simulink model "pocket_correlator"  (R2012b)
settings: Solver=ode45  StartTime=0.0  StopTime=10.0  RelTol=1e-3
libraries: xbsIndex_r4 x12697, casper_library_misc x57, simulink x17, casper_library_delays x14, dspsigops x12, xbsReplacements_r4 x10, xps_library x1
(part 4 of 125)

== system pocket_correlator/requant0 ==
  sync : Inport
  gain : Inport  Port=2
  in_even : Inport  Port=3
  in_odd : Inport  Port=4
  Constant{,1..3} (4 alike) : xbsIndex_r4/Constant  const=-1+1/(2^3)  gui_display_data_type=Fixed-point  arith_type=Signed (2's comp)  n_bits=4  bin_pt=3  preci_type=Single  exp_width=8  frac_width=24  explicit_period=on  period=1  equ=P=C  opselect=C  inp2=PCIN>>17  opr=+  inp1=P  carry=CIN  dbl_ovrd=off  block_type=constant
  Delay : xbsIndex_r4/Delay  rst=off  infoeditControl=Selection of Reset will increase slice count due to use of real FFs and instead of SRLs  en=off  latency=2  dbl_ovrd=off  reg_retiming=off  block_type=delay
  Delay1 : xbsIndex_r4/Delay  rst=off  infoeditControl=Selection of Reset will increase slice count due to use of real FFs and instead of SRLs  en=off  latency=3  dbl_ovrd=off  reg_retiming=off  block_type=delay
  Mult{,1..3} (4 alike) : xbsIndex_r4/Mult  precision=Full  arith_type="Signed  (2's comp)"  n_bits=16  bin_pt=14  quantization=Truncate  overflow=Wrap  en=off  latency=3  dbl_ovrd=off  use_behavioral_HDL=off  opt=Speed  use_embedded=on  optimum_pipeline=off  pipeline=on  use_rpm=on  placement_style=Triangular  block_type=mult
  Mux{,1..3} (4 alike) : xbsIndex_r4/Mux  inputs=2  en=off  latency=0  precision=Full  arith_type=Unsigned  n_bits=16  bin_pt=14  quantization=Truncate  overflow=Wrap  dbl_ovrd=off  block_type=mux
  Relational{,1..3} (4 alike) : xbsIndex_r4/Relational  mode=a<b  en=off  latency=2  dbl_ovrd=off  block_type=relational
  c_to_ri : casper_library_misc/c_to_ri  n_bits=18  bin_pt=17
  c_to_ri1 : casper_library_misc/c_to_ri  n_bits=18  bin_pt=17
  convert_of : Subsystem  AncestorBlock=casper_library_misc/convert_of  mask(convert_of){bit_width_i=34, binary_point_i=19, bit_width_o=4, binary_point_o=3, latency=2, overflow=Saturate, quantization=Round  (unbiased: even values)}
      mask prompts: bit_width_i "Bit Width In"; binary_point_i "Binary Point In"; bit_width_o "Bit Width Out"; binary_point_o "Binary Point Out"; overflow "Overflow Behaviour"; quantization "Quantization Behaviour"
      mask help:
      | Converts from one 2's complement bit-width
      | and/or binary point position to another.
      | Includes underflow/overflow indicator.
      mask init:
      | convert_of_init(gcb, ...
      |     'bit_width_i', bit_width_i, ...
      |     'binary_point_i', binary_point_i, ...
      |     'bit_width_o', bit_width_o, ...
      |     'binary_point_o', binary_point_o, ...
      |     'latency', latency, ...
      |     'overflow', overflow, ...
      |     'quantization', quantization);
      settings: AttributesFormatString=[34,19]->[4,3]
      mask TypeOptions overflow: Wrap | Saturate | Error
      mask TypeOptions quantization: Truncate | Round  (unbiased: +/- Inf) | Round  (unbiased: even values)
  convert_of1 : Subsystem  AncestorBlock=casper_library_misc/convert_of  mask(convert_of){bit_width_i=34, binary_point_i=19, bit_width_o=4, binary_point_o=3, latency=2, overflow=Saturate, quantization=Round  (unbiased: even values)}
      mask prompts: bit_width_i "Bit Width In"; binary_point_i "Binary Point In"; bit_width_o "Bit Width Out"; binary_point_o "Binary Point Out"; overflow "Overflow Behaviour"; quantization "Quantization Behaviour"
      mask help:
      | Converts from one 2's complement bit-width
      | and/or binary point position to another.
      | Includes underflow/overflow indicator.
      mask init: same as pocket_correlator/requant0/convert_of
      settings: AttributesFormatString=[34,19]->[4,3]
      mask TypeOptions overflow: Wrap | Saturate | Error
      mask TypeOptions quantization: Truncate | Round  (unbiased: +/- Inf) | Round  (unbiased: even values)
  convert_of2 : Subsystem  AncestorBlock=casper_library_misc/convert_of  mask(convert_of){bit_width_i=34, binary_point_i=19, bit_width_o=4, binary_point_o=3, latency=2, overflow=Saturate, quantization=Round  (unbiased: even values)}
      mask prompts: bit_width_i "Bit Width In"; binary_point_i "Binary Point In"; bit_width_o "Bit Width Out"; binary_point_o "Binary Point Out"; overflow "Overflow Behaviour"; quantization "Quantization Behaviour"
      mask help:
      | Converts from one 2's complement bit-width
      | and/or binary point position to another.
      | Includes underflow/overflow indicator.
      mask init: same as pocket_correlator/requant0/convert_of
      settings: AttributesFormatString=[34,19]->[4,3]
      mask TypeOptions overflow: Wrap | Saturate | Error
      mask TypeOptions quantization: Truncate | Round  (unbiased: +/- Inf) | Round  (unbiased: even values)
  convert_of3 : Subsystem  AncestorBlock=casper_library_misc/convert_of  mask(convert_of){bit_width_i=34, binary_point_i=19, bit_width_o=4, binary_point_o=3, latency=2, overflow=Saturate, quantization=Round  (unbiased: even values)}
      mask prompts: bit_width_i "Bit Width In"; binary_point_i "Binary Point In"; bit_width_o "Bit Width Out"; binary_point_o "Binary Point Out"; overflow "Overflow Behaviour"; quantization "Quantization Behaviour"
      mask help:
      | Converts from one 2's complement bit-width
      | and/or binary point position to another.
      | Includes underflow/overflow indicator.
      mask init: same as pocket_correlator/requant0/convert_of
      settings: AttributesFormatString=[34,19]->[4,3]
      mask TypeOptions overflow: Wrap | Saturate | Error
      mask TypeOptions quantization: Truncate | Round  (unbiased: +/- Inf) | Round  (unbiased: even values)
  ri_to_c : casper_library_misc/ri_to_c
  ri_to_c1 : casper_library_misc/ri_to_c
  sync_out : Outport
  out_even : Outport  Port=2
  out_odd : Outport  Port=3
  wires:
  sync/1 -> [sync_in], Delay1/1
  in_even/1 -> c_to_ri/1
  Mult/1 -> Relational/1, convert_of/1(din)
  Delay/1 -> sync_out/1
  Constant/1 -> Mux/3, Relational/2
  convert_of/1(dout) -> Mux/2
  Mult1/1 -> Relational1/1, convert_of1/1(din)
  Constant1/1 -> Relational1/2, Mux1/3
  convert_of1/1(dout) -> Mux1/2
  Mux/1 -> ri_to_c/1
  Mux1/1 -> ri_to_c/2
  ri_to_c/1 -> out_even/1
  in_odd/1 -> c_to_ri1/1
  Mult2/1 -> convert_of2/1(din), Relational2/1
  Constant2/1 -> Relational2/2, Mux2/3
  convert_of2/1(dout) -> Mux2/2
  Mult3/1 -> Relational3/1, convert_of3/1(din)
  Constant3/1 -> Mux3/3, Relational3/2
  convert_of3/1(dout) -> Mux3/2
  Mux2/1 -> ri_to_c1/1
  Mux3/1 -> ri_to_c1/2
  ri_to_c1/1 -> out_odd/1
  c_to_ri/1 -> Mult/2
  c_to_ri/2 -> Mult1/2
  gain/1 -> Mult2/1, Mult3/1, Mult1/1, Mult/1
  c_to_ri1/1 -> Mult2/2
  c_to_ri1/2 -> Mult3/2
  Delay1/1 -> Delay/1
  convert_of/2(of) -> [of0]
  convert_of1/2(of) -> [of1]
  convert_of2/2(of) -> [of2]
  convert_of3/2(of) -> [of3]
  Relational/1 -> Mux/1
  Relational1/1 -> Mux1/1
  Relational2/1 -> Mux2/1
  Relational3/1 -> Mux3/1

== system pocket_correlator/requant1 ==
  sync : Inport
  gain : Inport  Port=2
  in_even : Inport  Port=3
  in_odd : Inport  Port=4
  Constant{,1..3} (4 alike) : xbsIndex_r4/Constant  const=-1+1/(2^3)  gui_display_data_type=Fixed-point  arith_type=Signed (2's comp)  n_bits=4  bin_pt=3  preci_type=Single  exp_width=8  frac_width=24  explicit_period=on  period=1  equ=P=C  opselect=C  inp2=PCIN>>17  opr=+  inp1=P  carry=CIN  dbl_ovrd=off  block_type=constant
  Delay : xbsIndex_r4/Delay  rst=off  infoeditControl=Selection of Reset will increase slice count due to use of real FFs and instead of SRLs  en=off  latency=2  dbl_ovrd=off  reg_retiming=off  block_type=delay
  Delay1 : xbsIndex_r4/Delay  rst=off  infoeditControl=Selection of Reset will increase slice count due to use of real FFs and instead of SRLs  en=off  latency=3  dbl_ovrd=off  reg_retiming=off  block_type=delay
  Mult{,1..3} (4 alike) : xbsIndex_r4/Mult  precision=Full  arith_type="Signed  (2's comp)"  n_bits=16  bin_pt=14  quantization=Truncate  overflow=Wrap  en=off  latency=3  dbl_ovrd=off  use_behavioral_HDL=off  opt=Speed  use_embedded=on  optimum_pipeline=off  pipeline=on  use_rpm=on  placement_style=Triangular  block_type=mult
  Mux{,1..3} (4 alike) : xbsIndex_r4/Mux  inputs=2  en=off  latency=0  precision=Full  arith_type=Unsigned  n_bits=16  bin_pt=14  quantization=Truncate  overflow=Wrap  dbl_ovrd=off  block_type=mux
  Relational{,1..3} (4 alike) : xbsIndex_r4/Relational  mode=a<b  en=off  latency=2  dbl_ovrd=off  block_type=relational
  c_to_ri : casper_library_misc/c_to_ri  n_bits=18  bin_pt=17
  c_to_ri1 : casper_library_misc/c_to_ri  n_bits=18  bin_pt=17
  convert_of : Subsystem  AncestorBlock=casper_library_misc/convert_of  mask(convert_of){bit_width_i=34, binary_point_i=19, bit_width_o=4, binary_point_o=3, latency=2, overflow=Saturate, quantization=Round  (unbiased: even values)}
      mask prompts: bit_width_i "Bit Width In"; binary_point_i "Binary Point In"; bit_width_o "Bit Width Out"; binary_point_o "Binary Point Out"; overflow "Overflow Behaviour"; quantization "Quantization Behaviour"
      mask help:
      | Converts from one 2's complement bit-width
      | and/or binary point position to another.
      | Includes underflow/overflow indicator.
      mask init: same as pocket_correlator/requant0/convert_of
      settings: AttributesFormatString=[34,19]->[4,3]
      mask TypeOptions overflow: Wrap | Saturate | Error
      mask TypeOptions quantization: Truncate | Round  (unbiased: +/- Inf) | Round  (unbiased: even values)
  convert_of1 : Subsystem  AncestorBlock=casper_library_misc/convert_of  mask(convert_of){bit_width_i=34, binary_point_i=19, bit_width_o=4, binary_point_o=3, latency=2, overflow=Saturate, quantization=Round  (unbiased: even values)}
      mask prompts: bit_width_i "Bit Width In"; binary_point_i "Binary Point In"; bit_width_o "Bit Width Out"; binary_point_o "Binary Point Out"; overflow "Overflow Behaviour"; quantization "Quantization Behaviour"
      mask help:
      | Converts from one 2's complement bit-width
      | and/or binary point position to another.
      | Includes underflow/overflow indicator.
      mask init: same as pocket_correlator/requant0/convert_of
      settings: AttributesFormatString=[34,19]->[4,3]
      mask TypeOptions overflow: Wrap | Saturate | Error
      mask TypeOptions quantization: Truncate | Round  (unbiased: +/- Inf) | Round  (unbiased: even values)
  convert_of2 : Subsystem  AncestorBlock=casper_library_misc/convert_of  mask(convert_of){bit_width_i=34, binary_point_i=19, bit_width_o=4, binary_point_o=3, latency=2, overflow=Saturate, quantization=Round  (unbiased: even values)}
      mask prompts: bit_width_i "Bit Width In"; binary_point_i "Binary Point In"; bit_width_o "Bit Width Out"; binary_point_o "Binary Point Out"; overflow "Overflow Behaviour"; quantization "Quantization Behaviour"
      mask help:
      | Converts from one 2's complement bit-width
      | and/or binary point position to another.
      | Includes underflow/overflow indicator.
      mask init: same as pocket_correlator/requant0/convert_of
      settings: AttributesFormatString=[34,19]->[4,3]
      mask TypeOptions overflow: Wrap | Saturate | Error
      mask TypeOptions quantization: Truncate | Round  (unbiased: +/- Inf) | Round  (unbiased: even values)
  convert_of3 : Subsystem  AncestorBlock=casper_library_misc/convert_of  mask(convert_of){bit_width_i=34, binary_point_i=19, bit_width_o=4, binary_point_o=3, latency=2, overflow=Saturate, quantization=Round  (unbiased: even values)}
      mask prompts: bit_width_i "Bit Width In"; binary_point_i "Binary Point In"; bit_width_o "Bit Width Out"; binary_point_o "Binary Point Out"; overflow "Overflow Behaviour"; quantization "Quantization Behaviour"
      mask help:
      | Converts from one 2's complement bit-width
      | and/or binary point position to another.
      | Includes underflow/overflow indicator.
      mask init: same as pocket_correlator/requant0/convert_of
      settings: AttributesFormatString=[34,19]->[4,3]
      mask TypeOptions overflow: Wrap | Saturate | Error
      mask TypeOptions quantization: Truncate | Round  (unbiased: +/- Inf) | Round  (unbiased: even values)
  ri_to_c : casper_library_misc/ri_to_c
  ri_to_c1 : casper_library_misc/ri_to_c
  sync_out : Outport
  out_even : Outport  Port=2
  out_odd : Outport  Port=3
  wires:
  Relational3/1 -> Mux3/1
  Relational2/1 -> Mux2/1
  Relational1/1 -> Mux1/1
  Relational/1 -> Mux/1
  convert_of3/2(of) -> [of3]
  convert_of2/2(of) -> [of2]
  convert_of1/2(of) -> [of1]
  convert_of/2(of) -> [of0]
  Delay1/1 -> Delay/1
  c_to_ri1/2 -> Mult3/2
  c_to_ri1/1 -> Mult2/2
  gain/1 -> Mult/1, Mult1/1, Mult3/1, Mult2/1
  c_to_ri/2 -> Mult1/2
  c_to_ri/1 -> Mult/2
  ri_to_c1/1 -> out_odd/1
  Mux3/1 -> ri_to_c1/2
  Mux2/1 -> ri_to_c1/1
  convert_of3/1(dout) -> Mux3/2
  Constant3/1 -> Relational3/2, Mux3/3
  Mult3/1 -> convert_of3/1(din), Relational3/1
  convert_of2/1(dout) -> Mux2/2
  Constant2/1 -> Mux2/3, Relational2/2
  Mult2/1 -> Relational2/1, convert_of2/1(din)
  in_odd/1 -> c_to_ri1/1
  ri_to_c/1 -> out_even/1
  Mux1/1 -> ri_to_c/2
  Mux/1 -> ri_to_c/1
  convert_of1/1(dout) -> Mux1/2
  Constant1/1 -> Mux1/3, Relational1/2
  Mult1/1 -> convert_of1/1(din), Relational1/1
  convert_of/1(dout) -> Mux/2
  Constant/1 -> Relational/2, Mux/3
  Delay/1 -> sync_out/1
  Mult/1 -> convert_of/1(din), Relational/1
  in_even/1 -> c_to_ri/1
  sync/1 -> Delay1/1, [sync_in]

== system pocket_correlator/sync_ctrl ==
  sim_1 : Inport
  sim_2 : Inport  Port=2
  sim_3 : Inport  Port=3
  convert1_1 : DataTypeConversion  OutDataTypeStr=fixdt('ufix1_En0')  LockScale=on
  convert1_2 : DataTypeConversion  OutDataTypeStr=fixdt('ufix1_En0')  LockScale=on
  convert1_3 : DataTypeConversion  OutDataTypeStr=fixdt('ufix1_En0')  LockScale=on
  convert2_1 : DataTypeConversion  OutDataTypeStr=fixdt('ufix1_En0')  ConvertRealWorld=Stored Integer (SI)  LockScale=on
  convert2_2 : DataTypeConversion  OutDataTypeStr=fixdt('ufix1_En0')  ConvertRealWorld=Stored Integer (SI)  LockScale=on
  convert2_3 : DataTypeConversion  OutDataTypeStr=fixdt('ufix1_En0')  ConvertRealWorld=Stored Integer (SI)  LockScale=on
  gain_1 : Gain  Gain=4
  gain_2 : Gain  Gain=2
  gain_3 : Gain
  io_delay : xbsIndex_r4/Delay  rst=off  infoeditControl=Selection of Reset will increase slice count due to use of real FFs and instead of SRLs  en=off  latency=0  dbl_ovrd=off  reg_retiming=on  block_type=delay
  pocket_correlator_sync_ctrl_user_data_out : xbsIndex_r4/Gateway In  gui_display_data_type=Fixed-point  arith_type=Unsigned  n_bits=32  bin_pt=0  preci_type=Single  exp_width=8  frac_width=24  quantization="Round  (unbiased: +/- Inf)"  overflow=Saturate  period=1  dbl_ovrd=off  timing_constraint=None  locs_specified=off  LOCs={}  UseAsADC=off  ADCChannel='1'  inherit_from_input=off  hdl_port=on  block_type=gatewayin
  sim_add : Sum  Inputs=+++  OutDataTypeStr=uint32
  slice_enable_sync : xbsIndex_r4/Slice  nbits=1  boolean_output=on  mode=Lower Bit Location + Width  bit1=0  base1=MSB of Input  bit0=2  base0=LSB of Input  dbl_ovrd=off  block_type=slice
  slice_master_reset : xbsIndex_r4/Slice  nbits=1  boolean_output=on  mode=Lower Bit Location + Width  bit1=0  base1=MSB of Input  bit0=0  base0=LSB of Input  dbl_ovrd=off  block_type=slice
  slice_use_self_pps : xbsIndex_r4/Slice  nbits=1  boolean_output=on  mode=Lower Bit Location + Width  bit1=0  base1=MSB of Input  bit0=1  base0=LSB of Input  dbl_ovrd=off  block_type=slice
  in_enable_sync : Outport
  in_use_self_pps : Outport  Port=2
  in_master_reset : Outport  Port=3
  wires:
  pocket_correlator_sync_ctrl_user_data_out/1 -> io_delay/1
  sim_add/1 -> pocket_correlator_sync_ctrl_user_data_out/1
  sim_1/1 -> convert1_1/1
  convert1_1/1 -> convert2_1/1
  convert2_1/1 -> gain_1/1
  gain_1/1 -> sim_add/1
  io_delay/1 -> slice_enable_sync/1, slice_use_self_pps/1, slice_master_reset/1
  slice_enable_sync/1 -> in_enable_sync/1
  sim_2/1 -> convert1_2/1
  convert1_2/1 -> convert2_2/1
  convert2_2/1 -> gain_2/1
  gain_2/1 -> sim_add/2
  slice_use_self_pps/1 -> in_use_self_pps/1
  sim_3/1 -> convert1_3/1
  convert1_3/1 -> convert2_3/1
  convert2_3/1 -> gain_3/1
  gain_3/1 -> sim_add/3
  slice_master_reset/1 -> in_master_reset/1

== system pocket_correlator/acc_ctrl/edge_detect ==
  in : Inport
  Delay : xbsIndex_r4/Delay  rst=off  infoeditControl=Selection of Reset will increase slice count due to use of real FFs and instead of SRLs  en=off  latency=1  dbl_ovrd=off  reg_retiming=off  block_type=delay
      settings: xl_area=[0, 0, 0, 0, 0, 0, 0]
  Inverter : xbsIndex_r4/Inverter  en=off  latency=0  dbl_ovrd=off  block_type=inv
      settings: xl_area=[0, 0, 0, 0, 0, 0, 0]
  edge_op : xbsIndex_r4/Logical  logical_function=NOR  inputs=2  en=off  latency=0  precision=Full  arith_type=Unsigned  n_bits=8  bin_pt=2  align_bp=on  dbl_ovrd=off  block_type=logical
      settings: xl_area=[0, 0, 0, 0, 0, 0, 0]
  out : Outport
  wires:
  Inverter/1 -> edge_op/1
  edge_op/1 -> out/1
  in/1 -> Inverter/1, Delay/1
  Delay/1 -> edge_op/2

== system pocket_correlator/acc_ctrl/edge_detect1 ==
  in : Inport
  Delay : xbsIndex_r4/Delay  rst=off  infoeditControl=Selection of Reset will increase slice count due to use of real FFs and instead of SRLs  en=off  latency=1  dbl_ovrd=off  reg_retiming=off  block_type=delay
      settings: xl_area=[0, 0, 0, 0, 0, 0, 0]
  Inverter : xbsIndex_r4/Inverter  en=off  latency=0  dbl_ovrd=off  block_type=inv
      settings: xl_area=[0, 0, 0, 0, 0, 0, 0]
  edge_op : xbsIndex_r4/Logical  logical_function=NOR  inputs=2  en=off  latency=0  precision=Full  arith_type=Unsigned  n_bits=8  bin_pt=2  align_bp=on  dbl_ovrd=off  block_type=logical
      settings: xl_area=[0, 0, 0, 0, 0, 0, 0]
  out : Outport
  wires:
  Inverter/1 -> edge_op/1
  edge_op/1 -> out/1
  in/1 -> Inverter/1, Delay/1
  Delay/1 -> edge_op/2

== system pocket_correlator/acc_ctrl/edge_detect2 ==
  in : Inport
  Delay : xbsIndex_r4/Delay  rst=off  infoeditControl=Selection of Reset will increase slice count due to use of real FFs and instead of SRLs  en=off  latency=1  dbl_ovrd=off  reg_retiming=off  block_type=delay
      settings: xl_area=[0, 0, 0, 0, 0, 0, 0]
  Inverter : xbsIndex_r4/Inverter  en=off  latency=0  dbl_ovrd=off  block_type=inv
      settings: xl_area=[0, 0, 0, 0, 0, 0, 0]
  edge_op : xbsIndex_r4/Logical  logical_function=NOR  inputs=2  en=off  latency=0  precision=Full  arith_type=Unsigned  n_bits=8  bin_pt=2  align_bp=on  dbl_ovrd=off  block_type=logical
      settings: xl_area=[0, 0, 0, 0, 0, 0, 0]
  out : Outport
  wires:
  Inverter/1 -> edge_op/1
  edge_op/1 -> out/1
  in/1 -> Inverter/1, Delay/1
  Delay/1 -> edge_op/2

== system pocket_correlator/calc_adc_sum_sq/edge_detect2 ==
  in : Inport
  Delay : xbsIndex_r4/Delay  rst=off  infoeditControl=Selection of Reset will increase slice count due to use of real FFs and instead of SRLs  en=off  latency=1  dbl_ovrd=off  reg_retiming=off  block_type=delay
      settings: xl_area=[0, 0, 0, 0, 0, 0, 0]
  Inverter : xbsIndex_r4/Inverter  en=off  latency=0  dbl_ovrd=off  block_type=inv
      settings: xl_area=[0, 0, 0, 0, 0, 0, 0]
  edge_op : xbsIndex_r4/Logical  logical_function=AND  inputs=2  en=off  latency=0  precision=Full  arith_type=Unsigned  n_bits=8  bin_pt=2  align_bp=on  dbl_ovrd=off  block_type=logical
      settings: xl_area=[0, 0, 0, 0, 0, 0, 0]
  out : Outport
  wires:
  Inverter/1 -> edge_op/1
  edge_op/1 -> out/1
  in/1 -> Inverter/1, Delay/1
  Delay/1 -> edge_op/2

== system pocket_correlator/calc_adc_sum_sq4/edge_detect2 ==
  in : Inport
  Delay : xbsIndex_r4/Delay  rst=off  infoeditControl=Selection of Reset will increase slice count due to use of real FFs and instead of SRLs  en=off  latency=1  dbl_ovrd=off  reg_retiming=off  block_type=delay
      settings: xl_area=[0, 0, 0, 0, 0, 0, 0]
  Inverter : xbsIndex_r4/Inverter  en=off  latency=0  dbl_ovrd=off  block_type=inv
      settings: xl_area=[0, 0, 0, 0, 0, 0, 0]
  edge_op : xbsIndex_r4/Logical  logical_function=AND  inputs=2  en=off  latency=0  precision=Full  arith_type=Unsigned  n_bits=8  bin_pt=2  align_bp=on  dbl_ovrd=off  block_type=logical
      settings: xl_area=[0, 0, 0, 0, 0, 0, 0]
  out : Outport
  wires:
  Inverter/1 -> edge_op/1
  edge_op/1 -> out/1
  in/1 -> Inverter/1, Delay/1
  Delay/1 -> edge_op/2

== system pocket_correlator/dir_x0/aa ==
  a+bi : Inport
  c+di : Inport  Port=2
  new_acc : Inport  Port=3
  Counter : xbsIndex_r4/Counter  cnt_type=Free Running  cnt_to=Inf  operation=Up  start_count=0  cnt_by_val=1  arith_type=Unsigned  n_bits=chan_bits  bin_pt=0  load_pin=off  rst=on  en=on  explicit_period=off  period=1  dbl_ovrd=off  use_behavioral_HDL=off  implementation=Fabric  use_rpm=on  block_type=counter
      settings: xl_area=[0, 0, 0, 0, 0, 0, 0]
  Delay3 : xbsIndex_r4/Delay  rst=off  infoeditControl=Selection of Reset will increase slice count due to use of real FFs and instead of SRLs  en=off  latency=4  dbl_ovrd=off  reg_retiming=off  block_type=delay
      settings: xl_area=[0, 0, 0, 0, 0, 0, 0]
  Gateway Out{,1..3} (4 alike) : xbsIndex_r4/Gateway Out  inherit_from_input=off  hdl_port=on  timing_constraint=None  locs_specified=off  LOCs={}  UseAsDAC=off  DACChannel='1'  block_type=gatewayout
      settings: infoedit="Gateway out block.  Converts Xilinx fixed point inputs into ouputs of type Simulink integer, double, or fixed point.<P><P>Hardware notes:  In hardware these blocks become top level output ports or are discarded, depending on how they are configured."  xl_area=[0, 0, 0, 0, 0, 0, 0]  block_version=10.1.3
  Reinterpret : xbsIndex_r4/Reinterpret  force_arith_type=on  arith_type=Unsigned  force_bin_pt=on  bin_pt=0  block_type=reinterpret
      settings: infoedit="Changes signal type without altering the binary representation.   You can changed the signal between signed and unsigned, and relocate the binary point.<P><P>Hardware notes: In hardware this block costs nothing.<P><P>Example:  Suppose the input is 6 bits wide, signed, with 2 fractional bits, and the output is forced to unsigned with 0 fractional bits.  Then an input of -2.0 (1110.00 in binary 2's complement) becomes an output of 56 (111000 in binary)."  block_version=10.1.3
  Scope : Scope  NumInputPorts=4
      settings: YMin=-1~-1~-1~-1  YMax=1~1~1~1
  Terminator : Terminator
  c_to_ri : Subsystem  mask(Complex to Real-Imag){n_bits=4, bin_pt=3}
      mask prompts: n_bits "Bit Width"; bin_pt "Binary Point"
      mask help: Outputs real and imaginary components of a complex input.
      mask init:
      | annotation=sprintf('%d_%d r/i',n_bits,bin_pt);
      | set_param(gcb,'AttributesFormatString',annotation);
      settings: AttributesFormatString=4_3 r/i
      mask Help:
      | <pre>
      | Description::
      | 
      | Outputs real and imaginary components of a complex input.
      | Useful for simplifying interconnects.
      | See also: Real-Imag to Complex (ri_to_c)
      | 
      | Mask Parameters::
      | 
      | Bit Width (n_bits): Specifies the width of the real/imaginary components.
      | Assumed equal for both components.
      | 
      | Binary Point (bin_pt): Specifies the binary point location in the real/imaginary components.
      | Assumed equal for both components.
      | </pre>
  c_to_ri1 : Subsystem  mask(Complex to Real-Imag){n_bits=4, bin_pt=3}
      mask prompts: n_bits "Bit Width"; bin_pt "Binary Point"
      mask help: Outputs real and imaginary components of a complex input.
      mask init:
      | annotation=sprintf('%d_%d r/i',n_bits,bin_pt);
      | set_param(gcb,'AttributesFormatString',annotation);
      settings: AttributesFormatString=4_3 r/i
      mask Help:
      | <pre>
      | Description::
      | 
      | Outputs real and imaginary components of a complex input.
      | Useful for simplifying interconnects.
      | See also: Real-Imag to Complex (ri_to_c)
      | 
      | Mask Parameters::
      | 
      | Bit Width (n_bits): Specifies the width of the real/imaginary components.
      | Assumed equal for both components.
      | 
      | Binary Point (bin_pt): Specifies the binary point location in the real/imaginary components.
      | Assumed equal for both components.
      | </pre>
  cmult_dsp48e : Subsystem  AncestorBlock=casper_library_multipliers/cmult_dsp48e  mask(cmult_dsp48e){n_bits_a=4, bin_pt_a=3, n_bits_b=4, bin_pt_b=3, conjugated=on, full_precision=on, n_bits_c=37, bin_pt_c=34, quantization=Truncate, overflow=Wrap, cast_latency=0}
      mask prompts: n_bits_a "Bit width 'a'"; bin_pt_a "Binary point 'a'"; n_bits_b "Bit width 'b'"; bin_pt_b "Binary point 'b'"; conjugated "Conjugate"; full_precision "Full precision"; n_bits_c "Bit width out"; bin_pt_c "Binary point out"; cast_latency "Cast Latency"
      mask help:
      | Multiplies two complex numbers using 4 DSP48Es.
      | Conjugation is optional.
      |
      | Re{a} and Im{a} can be up to 25 bits.
      | Re{b} and Im{b} can be up to 18 bits.
      mask init:
      | cmult_dsp48e_init(gcb, ...
      |     'n_bits_a', n_bits_a, ...
      |     'bin_pt_a', bin_pt_a, ...
      |     'n_bits_b', n_bits_b, ...
      |     'bin_pt_b', bin_pt_b, ...
      |     'conjugated', conjugated, ...
      |     'full_precision', full_precision, ...
      |     'n_bits_c', n_bits_c, ...
      |     'bin_pt_c', bin_pt_c, ...
      |     'quantization', quantization, ...
      |     'overflow', overflow, ...
      |     'cast_latency', cast_latency);
      settings: AttributesFormatString=|
      | 4_3 * 4_3 ==> 9_6
      | Latency=4
      mask Callback full_precision:
      | full_precision = get_param(gcb, 'full_precision');
      | 
      | if strcmp(full_precision, 'on'),
      |     not_full_precision = 'off';
      | else
      |     not_full_precision = 'on';
      | end
      | 
      | set_param_state(gcb, 'n_bits_c', not_full_precision);
      | set_param_state(gcb, 'bin_pt_c', not_full_precision);
      | set_param_state(gcb, 'quantization', not_full_precision);
      | set_param_state(gcb, 'overflow', not_full_precision);
      | set_param_state(gcb, 'cast_latency', not_full_precision);
      mask TypeOptions quantization: Truncate | Round  (unbiased: +/- Inf) | Round  (unbiased: Even Values)
      mask TypeOptions overflow: Wrap | Saturate | Flag as error
  real : Subsystem  Tag=xps:bram  AncestorBlock=xps_library/Shared BRAM  mask{arith_type=Unsigned, addr_width=max(chan_bits,10), data_width=32, reg_prim_output=off, reg_core_output=off, optimization=Minimum_Area, data_bin_pt=0, init_vals=0, sample_rate=1}
      mask prompts: arith_type "Output Data Type"; addr_width "Address width"; data_width "Data Width"; reg_prim_output "Register Primitive Output"; reg_core_output "Register Core Output"; data_bin_pt "Data Binary Point"; init_vals "Initial values (simulation only)"; sample_rate "Sample rate"
      mask init:
      | shared_bram_mask;
      mask TypeOptions arith_type: Unsigned | Signed  (2's comp)
      mask TypeOptions data_width: 8 | 16 | 32 | 64 | 128
      mask TypeOptions optimization: Minimum_Area | Low_Power
  vacc_32bit : Subsystem  mask{n_chans=n_chans}
      mask prompts: n_chans "Number of channels"
      mask init:
      | chan_bits=ceil(log2(n_chans));
  wires:
  Reinterpret/1 -> real/2(data_in), Gateway Out1/1
  Counter/1 -> real/1(addr), Gateway Out/1
  vacc_32bit/2(valid) -> Counter/2, real/3(we), Gateway Out2/1
  Delay3/1 -> Counter/1, vacc_32bit/2(new_acc), Gateway Out3/1
  c+di/1 -> c_to_ri1/1(c)
  a+bi/1 -> c_to_ri/1(c)
  c_to_ri1/2(im) -> cmult_dsp48e/4(b_im)
  c_to_ri1/1(re) -> cmult_dsp48e/3(b_re)
  c_to_ri/2(im) -> cmult_dsp48e/2(a_im)
  c_to_ri/1(re) -> cmult_dsp48e/1(a_re)
  vacc_32bit/1(dout) -> Reinterpret/1
  new_acc/1 -> Delay3/1
  cmult_dsp48e/1(c_re) -> vacc_32bit/1(din)
  real/1(data_out) -> Terminator/1
  Gateway Out/1 -> Scope/1
  Gateway Out1/1 -> Scope/2
  Gateway Out2/1 -> Scope/3
  Gateway Out3/1 -> Scope/4

== system pocket_correlator/dir_x0/ab ==
  a+bi : Inport
  c+di : Inport  Port=2
  new_acc : Inport  Port=3
  Counter : xbsIndex_r4/Counter  cnt_type=Free Running  cnt_to=Inf  operation=Up  start_count=0  cnt_by_val=1  arith_type=Unsigned  n_bits=11  bin_pt=0  load_pin=off  rst=on  en=on  explicit_period=off  period=1  dbl_ovrd=off  use_behavioral_HDL=off  implementation=Fabric  use_rpm=on  block_type=counter
      settings: xl_area=[0, 0, 0, 0, 0, 0, 0]
  Delay3 : xbsIndex_r4/Delay  rst=off  infoeditControl=Selection of Reset will increase slice count due to use of real FFs and instead of SRLs  en=off  latency=4  dbl_ovrd=off  reg_retiming=off  block_type=delay
      settings: xl_area=[0, 0, 0, 0, 0, 0, 0]
  Reinterpret : xbsIndex_r4/Reinterpret  force_arith_type=on  arith_type=Unsigned  force_bin_pt=on  bin_pt=0  block_type=reinterpret
      settings: infoedit="Changes signal type without altering the binary representation.   You can changed the signal between signed and unsigned, and relocate the binary point.<P><P>Hardware notes: In hardware this block costs nothing.<P><P>Example:  Suppose the input is 6 bits wide, signed, with 2 fractional bits, and the output is forced to unsigned with 0 fractional bits.  Then an input of -2.0 (1110.00 in binary 2's complement) becomes an output of 56 (111000 in binary)."  block_version=10.1.3
  Reinterpret1 : xbsIndex_r4/Reinterpret  force_arith_type=on  arith_type=Unsigned  force_bin_pt=on  bin_pt=0  block_type=reinterpret
      settings: infoedit="Changes signal type without altering the binary representation.   You can changed the signal between signed and unsigned, and relocate the binary point.<P><P>Hardware notes: In hardware this block costs nothing.<P><P>Example:  Suppose the input is 6 bits wide, signed, with 2 fractional bits, and the output is forced to unsigned with 0 fractional bits.  Then an input of -2.0 (1110.00 in binary 2's complement) becomes an output of 56 (111000 in binary)."  block_version=10.1.3
  c_to_ri : Subsystem  mask(Complex to Real-Imag){n_bits=4, bin_pt=3}
      mask prompts: n_bits "Bit Width"; bin_pt "Binary Point"
      mask help: Outputs real and imaginary components of a complex input.
      mask init:
      | annotation=sprintf('%d_%d r/i',n_bits,bin_pt);
      | set_param(gcb,'AttributesFormatString',annotation);
      settings: AttributesFormatString=4_3 r/i
      mask Help:
      | <pre>
      | Description::
      | 
      | Outputs real and imaginary components of a complex input.
      | Useful for simplifying interconnects.
      | See also: Real-Imag to Complex (ri_to_c)
      | 
      | Mask Parameters::
      | 
      | Bit Width (n_bits): Specifies the width of the real/imaginary components.
      | Assumed equal for both components.
      | 
      | Binary Point (bin_pt): Specifies the binary point location in the real/imaginary components.
      | Assumed equal for both components.
      | </pre>
  c_to_ri1 : Subsystem  mask(Complex to Real-Imag){n_bits=4, bin_pt=3}
      mask prompts: n_bits "Bit Width"; bin_pt "Binary Point"
      mask help: Outputs real and imaginary components of a complex input.
      mask init:
      | annotation=sprintf('%d_%d r/i',n_bits,bin_pt);
      | set_param(gcb,'AttributesFormatString',annotation);
      settings: AttributesFormatString=4_3 r/i
      mask Help:
      | <pre>
      | Description::
      | 
      | Outputs real and imaginary components of a complex input.
      | Useful for simplifying interconnects.
      | See also: Real-Imag to Complex (ri_to_c)
      | 
      | Mask Parameters::
      | 
      | Bit Width (n_bits): Specifies the width of the real/imaginary components.
      | Assumed equal for both components.
      | 
      | Binary Point (bin_pt): Specifies the binary point location in the real/imaginary components.
      | Assumed equal for both components.
      | </pre>
  cmult_dsp48e : Subsystem  AncestorBlock=casper_library_multipliers/cmult_dsp48e  mask(cmult_dsp48e){n_bits_a=4, bin_pt_a=3, n_bits_b=4, bin_pt_b=3, conjugated=on, full_precision=on, n_bits_c=37, bin_pt_c=34, quantization=Truncate, overflow=Wrap, cast_latency=0}
      mask prompts: n_bits_a "Bit width 'a'"; bin_pt_a "Binary point 'a'"; n_bits_b "Bit width 'b'"; bin_pt_b "Binary point 'b'"; conjugated "Conjugate"; full_precision "Full precision"; n_bits_c "Bit width out"; bin_pt_c "Binary point out"; cast_latency "Cast Latency"
      mask help:
      | Multiplies two complex numbers using 4 DSP48Es.
      | Conjugation is optional.
      |
      | Re{a} and Im{a} can be up to 25 bits.
      | Re{b} and Im{b} can be up to 18 bits.
      mask init: same as pocket_correlator/dir_x0/aa/cmult_dsp48e
      settings: AttributesFormatString=|
      | 4_3 * 4_3 ==> 9_6
      | Latency=4
      mask Callback full_precision:
      | full_precision = get_param(gcb, 'full_precision');
      | 
      | if strcmp(full_precision, 'on'),
      |     not_full_precision = 'off';
      | else
      |     not_full_precision = 'on';
      | end
      | 
      | set_param_state(gcb, 'n_bits_c', not_full_precision);
      | set_param_state(gcb, 'bin_pt_c', not_full_precision);
      | set_param_state(gcb, 'quantization', not_full_precision);
      | set_param_state(gcb, 'overflow', not_full_precision);
      | set_param_state(gcb, 'cast_latency', not_full_precision);
      mask TypeOptions quantization: Truncate | Round  (unbiased: +/- Inf) | Round  (unbiased: Even Values)
      mask TypeOptions overflow: Wrap | Saturate | Flag as error
  imag : Subsystem  Tag=xps:bram  AncestorBlock=xps_library/Shared BRAM  mask{arith_type=Unsigned, addr_width=max(chan_bits,10), data_width=32, reg_prim_output=off, reg_core_output=off, optimization=Minimum_Area, data_bin_pt=0, init_vals=0, sample_rate=1}
      mask prompts: arith_type "Output Data Type"; addr_width "Address width"; data_width "Data Width"; reg_prim_output "Register Primitive Output"; reg_core_output "Register Core Output"; data_bin_pt "Data Binary Point"; init_vals "Initial values (simulation only)"; sample_rate "Sample rate"
      mask init:
      | shared_bram_mask;
      mask TypeOptions arith_type: Unsigned | Signed  (2's comp)
      mask TypeOptions data_width: 8 | 16 | 32 | 64 | 128
      mask TypeOptions optimization: Minimum_Area | Low_Power
  real : Subsystem  Tag=xps:bram  AncestorBlock=xps_library/Shared BRAM  mask{arith_type=Unsigned, addr_width=max(chan_bits,10), data_width=32, reg_prim_output=off, reg_core_output=off, optimization=Minimum_Area, data_bin_pt=0, init_vals=0, sample_rate=1}
      mask prompts: arith_type "Output Data Type"; addr_width "Address width"; data_width "Data Width"; reg_prim_output "Register Primitive Output"; reg_core_output "Register Core Output"; data_bin_pt "Data Binary Point"; init_vals "Initial values (simulation only)"; sample_rate "Sample rate"
      mask init:
      | shared_bram_mask;
      mask TypeOptions arith_type: Unsigned | Signed  (2's comp)
      mask TypeOptions data_width: 8 | 16 | 32 | 64 | 128
      mask TypeOptions optimization: Minimum_Area | Low_Power
  vacc_0 : Subsystem  mask{n_chans=n_chans}
      mask prompts: n_chans "Number of channels"
      mask init:
      | chan_bits=ceil(log2(n_chans));
  vacc_1 : Subsystem  mask{n_chans=n_chans}
      mask prompts: n_chans "Number of channels"
      mask init:
      | chan_bits=ceil(log2(n_chans));
  wires:
  Counter/1 -> real/1(addr), imag/1(addr)
  vacc_1/1(dout) -> Reinterpret1/1
  Reinterpret1/1 -> imag/2(data_in)
  vacc_1/2(valid) -> imag/3(we)
  Reinterpret/1 -> real/2(data_in)
  vacc_0/2(valid) -> real/3(we), Counter/2
  vacc_0/1(dout) -> Reinterpret/1
  new_acc/1 -> Delay3/1
  Delay3/1 -> vacc_0/2(new_acc), Counter/1, vacc_1/2(new_acc)
  c+di/1 -> c_to_ri1/1(c)
  a+bi/1 -> c_to_ri/1(c)
  c_to_ri1/2(im) -> cmult_dsp48e/4(b_im)
  c_to_ri1/1(re) -> cmult_dsp48e/3(b_re)
  c_to_ri/2(im) -> cmult_dsp48e/2(a_im)
  c_to_ri/1(re) -> cmult_dsp48e/1(a_re)
  cmult_dsp48e/2(c_im) -> vacc_1/1(din)
  cmult_dsp48e/1(c_re) -> vacc_0/1(din)

== system pocket_correlator/dir_x0/bb ==
  a+bi : Inport
  c+di : Inport  Port=2
  new_acc : Inport  Port=3
  Counter : xbsIndex_r4/Counter  cnt_type=Free Running  cnt_to=Inf  operation=Up  start_count=0  cnt_by_val=1  arith_type=Unsigned  n_bits=chan_bits  bin_pt=0  load_pin=off  rst=on  en=on  explicit_period=off  period=1  dbl_ovrd=off  use_behavioral_HDL=off  implementation=Fabric  use_rpm=on  block_type=counter
      settings: xl_area=[0, 0, 0, 0, 0, 0, 0]
  Delay3 : xbsIndex_r4/Delay  rst=off  infoeditControl=Selection of Reset will increase slice count due to use of real FFs and instead of SRLs  en=off  latency=4  dbl_ovrd=off  reg_retiming=off  block_type=delay
      settings: xl_area=[0, 0, 0, 0, 0, 0, 0]
  Gateway Out{,1..3} (4 alike) : xbsIndex_r4/Gateway Out  inherit_from_input=off  hdl_port=on  timing_constraint=None  locs_specified=off  LOCs={}  UseAsDAC=off  DACChannel='1'  block_type=gatewayout
      settings: infoedit="Gateway out block.  Converts Xilinx fixed point inputs into ouputs of type Simulink integer, double, or fixed point.<P><P>Hardware notes:  In hardware these blocks become top level output ports or are discarded, depending on how they are configured."  xl_area=[0, 0, 0, 0, 0, 0, 0]  block_version=10.1.3
  Reinterpret : xbsIndex_r4/Reinterpret  force_arith_type=on  arith_type=Unsigned  force_bin_pt=on  bin_pt=0  block_type=reinterpret
      settings: infoedit="Changes signal type without altering the binary representation.   You can changed the signal between signed and unsigned, and relocate the binary point.<P><P>Hardware notes: In hardware this block costs nothing.<P><P>Example:  Suppose the input is 6 bits wide, signed, with 2 fractional bits, and the output is forced to unsigned with 0 fractional bits.  Then an input of -2.0 (1110.00 in binary 2's complement) becomes an output of 56 (111000 in binary)."  block_version=10.1.3
  Scope : Scope  NumInputPorts=4
      settings: YMin=-1~-1~-1~-1  YMax=1~1~1~1
  Terminator : Terminator
  c_to_ri : Subsystem  mask(Complex to Real-Imag){n_bits=4, bin_pt=3}
      mask prompts: n_bits "Bit Width"; bin_pt "Binary Point"
      mask help: Outputs real and imaginary components of a complex input.
      mask init:
      | annotation=sprintf('%d_%d r/i',n_bits,bin_pt);
      | set_param(gcb,'AttributesFormatString',annotation);
      settings: AttributesFormatString=4_3 r/i
      mask Help:
      | <pre>
      | Description::
      | 
      | Outputs real and imaginary components of a complex input.
      | Useful for simplifying interconnects.
      | See also: Real-Imag to Complex (ri_to_c)
      | 
      | Mask Parameters::
      | 
      | Bit Width (n_bits): Specifies the width of the real/imaginary components.
      | Assumed equal for both components.
      | 
      | Binary Point (bin_pt): Specifies the binary point location in the real/imaginary components.
      | Assumed equal for both components.
      | </pre>
  c_to_ri1 : Subsystem  mask(Complex to Real-Imag){n_bits=4, bin_pt=3}
      mask prompts: n_bits "Bit Width"; bin_pt "Binary Point"
      mask help: Outputs real and imaginary components of a complex input.
      mask init:
      | annotation=sprintf('%d_%d r/i',n_bits,bin_pt);
      | set_param(gcb,'AttributesFormatString',annotation);
      settings: AttributesFormatString=4_3 r/i
      mask Help:
      | <pre>
      | Description::
      | 
      | Outputs real and imaginary components of a complex input.
      | Useful for simplifying interconnects.
      | See also: Real-Imag to Complex (ri_to_c)
      | 
      | Mask Parameters::
      | 
      | Bit Width (n_bits): Specifies the width of the real/imaginary components.
      | Assumed equal for both components.
      | 
      | Binary Point (bin_pt): Specifies the binary point location in the real/imaginary components.
      | Assumed equal for both components.
      | </pre>
  cmult_dsp48e : Subsystem  AncestorBlock=casper_library_multipliers/cmult_dsp48e  mask(cmult_dsp48e){n_bits_a=4, bin_pt_a=3, n_bits_b=4, bin_pt_b=3, conjugated=on, full_precision=on, n_bits_c=37, bin_pt_c=34, quantization=Truncate, overflow=Wrap, cast_latency=0}
      mask prompts: n_bits_a "Bit width 'a'"; bin_pt_a "Binary point 'a'"; n_bits_b "Bit width 'b'"; bin_pt_b "Binary point 'b'"; conjugated "Conjugate"; full_precision "Full precision"; n_bits_c "Bit width out"; bin_pt_c "Binary point out"; cast_latency "Cast Latency"
      mask help:
      | Multiplies two complex numbers using 4 DSP48Es.
      | Conjugation is optional.
      |
      | Re{a} and Im{a} can be up to 25 bits.
      | Re{b} and Im{b} can be up to 18 bits.
      mask init: same as pocket_correlator/dir_x0/aa/cmult_dsp48e
      settings: AttributesFormatString=|
      | 4_3 * 4_3 ==> 9_6
      | Latency=4
      mask Callback full_precision:
      | full_precision = get_param(gcb, 'full_precision');
      | 
      | if strcmp(full_precision, 'on'),
      |     not_full_precision = 'off';
      | else
      |     not_full_precision = 'on';
      | end
      | 
      | set_param_state(gcb, 'n_bits_c', not_full_precision);
      | set_param_state(gcb, 'bin_pt_c', not_full_precision);
      | set_param_state(gcb, 'quantization', not_full_precision);
      | set_param_state(gcb, 'overflow', not_full_precision);
      | set_param_state(gcb, 'cast_latency', not_full_precision);
      mask TypeOptions quantization: Truncate | Round  (unbiased: +/- Inf) | Round  (unbiased: Even Values)
      mask TypeOptions overflow: Wrap | Saturate | Flag as error
  real : Subsystem  Tag=xps:bram  AncestorBlock=xps_library/Shared BRAM  mask{arith_type=Unsigned, addr_width=max(chan_bits,10), data_width=32, reg_prim_output=off, reg_core_output=off, optimization=Minimum_Area, data_bin_pt=0, init_vals=0, sample_rate=1}
      mask prompts: arith_type "Output Data Type"; addr_width "Address width"; data_width "Data Width"; reg_prim_output "Register Primitive Output"; reg_core_output "Register Core Output"; data_bin_pt "Data Binary Point"; init_vals "Initial values (simulation only)"; sample_rate "Sample rate"
      mask init:
      | shared_bram_mask;
      mask TypeOptions arith_type: Unsigned | Signed  (2's comp)
      mask TypeOptions data_width: 8 | 16 | 32 | 64 | 128
      mask TypeOptions optimization: Minimum_Area | Low_Power
  vacc_32bit : Subsystem  mask{n_chans=n_chans}
      mask prompts: n_chans "Number of channels"
      mask init:
      | chan_bits=ceil(log2(n_chans));
  wires:
  Gateway Out3/1 -> Scope/4
  Gateway Out2/1 -> Scope/3
  Gateway Out1/1 -> Scope/2
  Gateway Out/1 -> Scope/1
  real/1(data_out) -> Terminator/1
  cmult_dsp48e/1(c_re) -> vacc_32bit/1(din)
  new_acc/1 -> Delay3/1
  vacc_32bit/1(dout) -> Reinterpret/1
  c_to_ri/1(re) -> cmult_dsp48e/1(a_re)
  c_to_ri/2(im) -> cmult_dsp48e/2(a_im)
  c_to_ri1/1(re) -> cmult_dsp48e/3(b_re)
  c_to_ri1/2(im) -> cmult_dsp48e/4(b_im)
  a+bi/1 -> c_to_ri/1(c)
  c+di/1 -> c_to_ri1/1(c)
  Delay3/1 -> Gateway Out3/1, vacc_32bit/2(new_acc), Counter/1
  vacc_32bit/2(valid) -> Gateway Out2/1, real/3(we), Counter/2
  Counter/1 -> Gateway Out/1, real/1(addr)
  Reinterpret/1 -> Gateway Out1/1, real/2(data_in)
